simulink model "torque_control_motor_sm"  (R2023b)
settings: Solver=FixedStepAuto  StartTime=0.0  StopTime=inf  RelTol=1e-3  EnableMultiTasking=on
undefined symbols (not defined in the file): G_v
libraries: mbedblockslib x6, cstblocks x3, stm_qeplib x1
settings Model: ExtModeTrigDuration=10  Creator=miche  LastModifiedBy=miche
settings OptimizationCC: EnhancedBackFolding=on  PassReuseOutputArgsAs=Individual arguments  ZeroExternalMemoryAtStartup=off  ZeroInternalMemoryAtStartup=off  MaxStackSize=64  OptimizeBlockOrder=speed  DifferentSizesBufferReuse=on  OptimizationCustomize=off  EfficientTunableParamExpr=on
settings DebuggingCC: ParameterTunabilityLossMsg=error
settings HardwareCC: ProdBitPerPointer=32  ProdBitPerSizeT=32  ProdBitPerPtrDiffT=32  ProdLargestAtomicInteger=Long  ProdLargestAtomicFloat=Double  ProdWordSize=32  ProdLongLongMode=on  ProdHWDeviceType=ARM Compatible->ARM Cortex
settings SFSimCC: MATLABDynamicMemAlloc=off
settings RTWCC: Description=Embedded Coder  SystemTargetFile=ert.tlc  HardwareBoard=STM32 Nucleo F401RE  TemplateMakefile=ert_default_tmf  Toolchain=GNU Tools for ARM Embedded Processors
settings CodeAppCC: ForceParamTrailComments=on  IgnoreCustomStorageClasses=off  OperatorAnnotations=on  SimulinkDataObjDesc=on  SFDataObjDesc=on  InsertBlockDesc=on
settings ERTTargetCC: ExtModeTransport=3  ExtModeStaticAlloc=on  ExtModeStaticAllocSize=2000  ExtModeMexFile=ext_xcp  ExtModeIntrfLevel=Level2 - Open

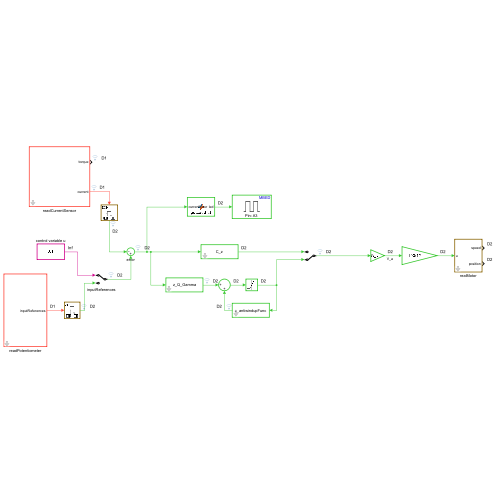
[thumbnail: Simulink's stored preview of the top-level diagram]
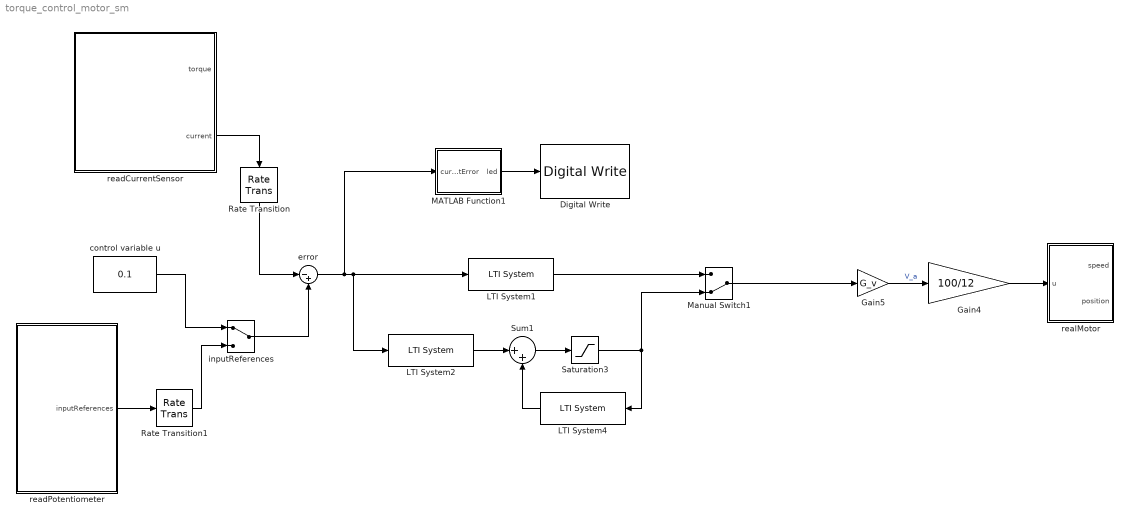
== system torque_control_motor_sm ==
  Digital Write : mbedblockslib/Digital Write  Pin=A3  Direction=output
      settings: LibrarySourceBlock=stmnucleorootlib/Common/Digital Write
  Gain4 : Gain  Gain=100/12
  Gain5 : Gain  Gain=G_v
  LTI System1 : cstblocks/LTI System  sys=C_z  IC=[]  PadeOrder=0
  LTI System2 : cstblocks/LTI System  sys=z_Q_Gamma  IC=[]  PadeOrder=0
  LTI System4 : cstblocks/LTI System  sys=z_antiwindupFunc  IC=[]  PadeOrder=0
  MATLAB Function1 : MATLAB Function  TreatAsAtomicUnit=on
  Manual Switch1 : ManualSwitch  CurrentSetting=0
  Rate Transition : RateTransition
  Rate Transition1 : RateTransition
  Saturation3 : Saturate  UpperLimit=12  LowerLimit=-12
  Sum1 : Sum  Inputs=|++
  control variable u : Constant  Value=0.1
  error : Sum  Inputs=|-+
  inputReferences : ManualSwitch
  readCurrentSensor : Subsystem  mask{alpha=0.9}
  readPotentiometer : Subsystem  mask{alpha=0.9}
  realMotor : Subsystem  mask{Ts=0.005}
      mask prompts: Ts "sample_time"
  wires:
  Gain5/1 -> Gain4/1  "V_a"
  inputReferences/1 -> error/2
  error/1 -> MATLAB Function1/1(currentError), LTI System2/1, LTI System1/1
  MATLAB Function1/1(led) -> Digital Write/1
  control variable u/1 -> inputReferences/1
  Gain4/1 -> realMotor/1(u)
  readPotentiometer/1(inputReferences) -> Rate Transition1/1
  readCurrentSensor/2(current) -> Rate Transition/1
  LTI System4/1 -> Sum1/2
  Saturation3/1 -> LTI System4/1, Manual Switch1/2
  LTI System2/1 -> Sum1/1
  Manual Switch1/1 -> Gain5/1
  Sum1/1 -> Saturation3/1
  LTI System1/1 -> Manual Switch1/1
  Rate Transition/1 -> error/1
  Rate Transition1/1 -> inputReferences/2

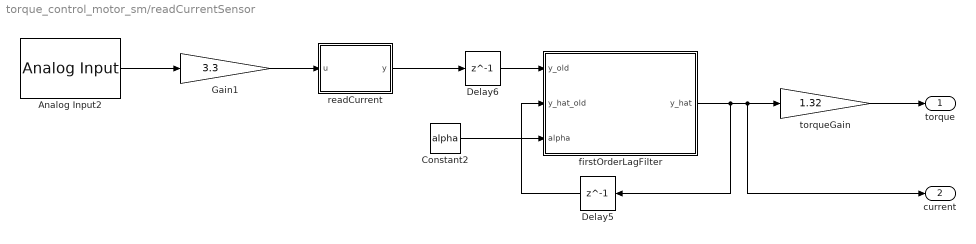
== system torque_control_motor_sm/readCurrentSensor ==
  Analog Input2 : mbedblockslib/Analog Input  Pin=A5  ReadResultsOnly=off  ConversionTriggerSource=Software  ExternalTriggerType=uint32( 0 )  OutputDataType=double  EnableConversionCompleteNotify=off  EnableOuputStatus=off  SampleTime=0.005/20
      settings: LibrarySourceBlock=stmnucleorootlib/Common/Analog Input
  Constant2 : Constant  Value=alpha
  Delay5 : Delay  DelayLength=1  InitialCondition=0
  Delay6 : Delay  DelayLength=1  InitialCondition=0
  Gain1 : Gain  Gain=3.3
  firstOrderLagFilter : MATLAB Function  TreatAsAtomicUnit=on
  readCurrent : MATLAB Function  TreatAsAtomicUnit=on
  torqueGain : Gain  Gain=1.32
  torque : Outport
  current : Outport  Port=2
  wires:
  Constant2/1 -> firstOrderLagFilter/3(alpha)
  firstOrderLagFilter/1(y_hat) -> current/1, torqueGain/1, Delay5/1
  torqueGain/1 -> torque/1
  Gain1/1 -> readCurrent/1(u)
  Analog Input2/1 -> Gain1/1
  readCurrent/1(y) -> Delay6/1
  Delay5/1 -> firstOrderLagFilter/2(y_hat_old)
  Delay6/1 -> firstOrderLagFilter/1(y_old)

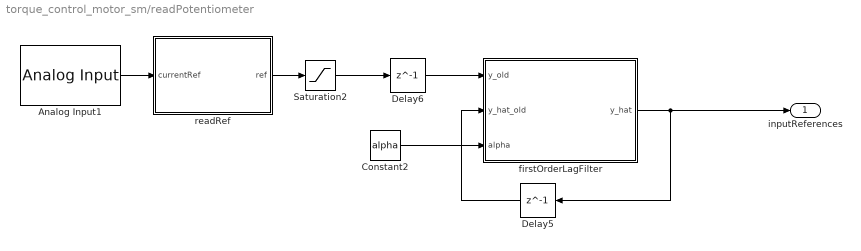
== system torque_control_motor_sm/readPotentiometer ==
  Analog Input1 : mbedblockslib/Analog Input  Pin=A4  ReadResultsOnly=off  ConversionTriggerSource=Software  ExternalTriggerType=uint32( 0 )  OutputDataType=double  EnableConversionCompleteNotify=off  EnableOuputStatus=off  SampleTime=0.005/20
      settings: LibrarySourceBlock=stmnucleorootlib/Common/Analog Input
  Constant2 : Constant  Value=alpha
  Delay5 : Delay  DelayLength=1  InitialCondition=0
  Delay6 : Delay  DelayLength=1  InitialCondition=0
  Saturation2 : Saturate  UpperLimit=0.25  LowerLimit=0
  firstOrderLagFilter : MATLAB Function  TreatAsAtomicUnit=on
  readRef : MATLAB Function  TreatAsAtomicUnit=on
  inputReferences : Outport
  wires:
  Saturation2/1 -> Delay6/1
  Delay6/1 -> firstOrderLagFilter/1(y_old)
  readRef/1(ref) -> Saturation2/1
  Constant2/1 -> firstOrderLagFilter/3(alpha)
  Delay5/1 -> firstOrderLagFilter/2(y_hat_old)
  firstOrderLagFilter/1(y_hat) -> inputReferences/1, Delay5/1
  Analog Input1/1 -> readRef/1(currentRef)

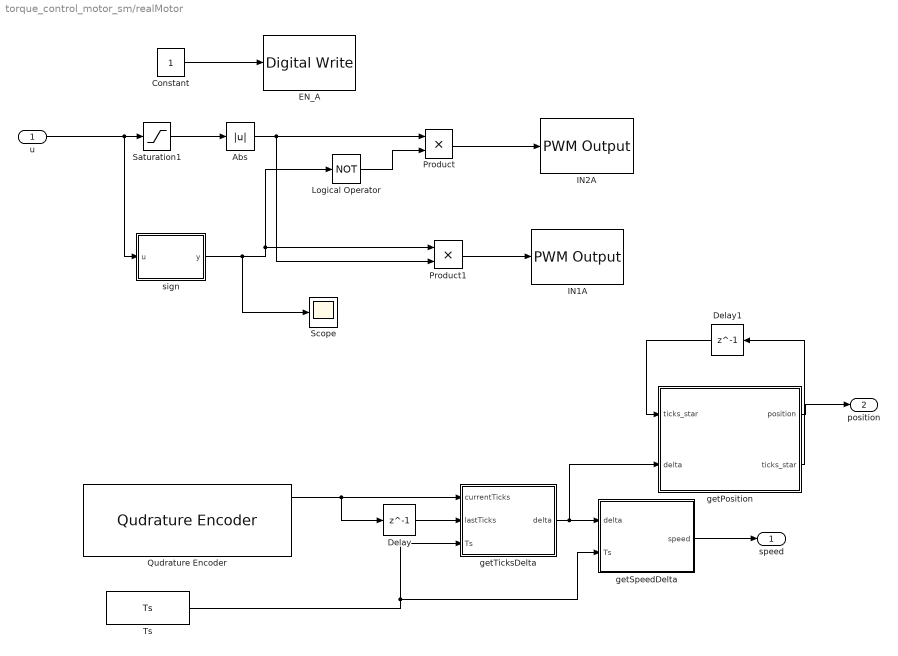
== system torque_control_motor_sm/realMotor ==
  u : Inport
  Abs : Abs  SaturateOnIntegerOverflow=off
  Constant : Constant
  Delay : Delay  DelayLength=1  InitialCondition=0
  Delay1 : Delay  DelayLength=1  InitialCondition=0
  EN_A : mbedblockslib/Digital Write  Pin=2  Direction=output
      settings: LibrarySourceBlock=stmnucleorootlib/Common/Digital Write
  IN1A : mbedblockslib/PWM Output  Pin=5  EnableInputFrequency=off  InitialFrequency=2000  InitialDutyCycle=50  NotificationType=None
      settings: LibrarySourceBlock=stmnucleorootlib/Common/PWM Output
  IN2A : mbedblockslib/PWM Output  Pin=4  EnableInputFrequency=off  InitialFrequency=2000  InitialDutyCycle=50  NotificationType=None
      settings: LibrarySourceBlock=stmnucleorootlib/Common/PWM Output
  Logical Operator : Logic  Operator=NOT  AllPortsSameDT=off  OutDataTypeStr=boolean
  Product : Product
  Product1 : Product
  Qudrature Encoder : stm_qeplib/Qudrature Encoder  SampleTime=0.005
  Saturation1 : Saturate  UpperLimit=100  LowerLimit=-100
  Scope : Scope
  Ts : Constant  Value=Ts
  getPosition : MATLAB Function  TreatAsAtomicUnit=on
  getSpeedDelta : MATLAB Function  TreatAsAtomicUnit=on
  getTicksDelta : MATLAB Function  TreatAsAtomicUnit=on
  sign : MATLAB Function  TreatAsAtomicUnit=on
  speed : Outport
  position : Outport  Port=2
  wires:
  sign/1(y) -> Scope/1, Product1/1, Logical Operator/1
  Ts/1 -> getSpeedDelta/2(Ts), getTicksDelta/3(Ts)
  Qudrature Encoder/1 -> Delay/1, getTicksDelta/1(currentTicks)
  Delay1/1 -> getPosition/1("ticks_star ")
  Constant/1 -> EN_A/1
  getPosition/2(ticks_star) -> Delay1/1
  getTicksDelta/1(delta) -> getPosition/2(delta), getSpeedDelta/1(delta)
  Abs/1 -> Product1/2, Product/1
  Product/1 -> IN2A/1
  Logical Operator/1 -> Product/2
  Product1/1 -> IN1A/1
  Delay/1 -> getTicksDelta/2(lastTicks)
  Saturation1/1 -> Abs/1
  getPosition/1(position) -> position/1
  u/1 -> sign/1(u), Saturation1/1
  getSpeedDelta/1(speed) -> speed/1

== matlab function torque_control_motor_sm/realMotor/getPosition ==
  data: ticks_star input; delta input; position output; ticks_star output
function [position,ticks_star] = getPosition(ticks_star, delta)
    ticks_star=double(ticks_star + delta);
    completeTheta=2*pi*ticks_star/(8400);
    position=completeTheta
    %position=sign(completeTheta)*mod(abs(completeTheta), 2*pi)
end

== matlab function torque_control_motor_sm/realMotor/getSpeedDelta ==
  data: delta input; speed output; Ts input
function speed=getSpeedDelta(delta,Ts)
speed=delta * 60/ (8400*Ts);
end

== matlab function torque_control_motor_sm/readCurrentSensor/firstOrderLagFilter ==
  data: y_old input; y_hat output; y_hat_old input; alpha input
function y_hat = firstOrderLagFilter(y_old, y_hat_old, alpha)
    y_hat= (alpha *y_hat_old) + ((1-alpha)* y_old)
end

== matlab function torque_control_motor_sm/readCurrentSensor/readCurrent ==
  data: u input; y output
function y = readCurrent(u)


y=(u-2.5-0.070)/0.185

== matlab function torque_control_motor_sm/MATLAB Function1 ==
  data: currentError input; led output
function led = getLedStat(currentError) 

    if abs(currentError) < 0.03
        led = true;
    else
        led = false;
    end


end

== matlab function torque_control_motor_sm/realMotor/getTicksDelta ==
  data: currentTicks input; delta output; lastTicks input; Ts input
function delta = getTicksDelta(currentTicks,lastTicks, Ts)

currentTicks=double(currentTicks);
lastTicks=double(lastTicks);

if abs(currentTicks -lastTicks) <= ceil(12600*Ts)
    delta= currentTicks - lastTicks;
else
    if lastTicks > currentTicks
        delta= currentTicks + 2^16 -1 - lastTicks;
    else
        delta= currentTicks - 2^16 +1 - lastTicks;
    end
end

end

== matlab function torque_control_motor_sm/realMotor/sign ==
  data: u input; y output
function y = sign(u)
if u >0
    y=1;
else
   y=0;
end

== matlab function torque_control_motor_sm/readPotentiometer/firstOrderLagFilter ==
  data: y_old input; y_hat output; y_hat_old input; alpha input
function y_hat = firstOrderLagFilter(y_old, y_hat_old, alpha)
    y_hat= (alpha *y_hat_old) + ((1-alpha)* y_old)
end

== matlab function torque_control_motor_sm/readPotentiometer/readRef ==
  data: currentRef input; ref output
function ref= getRef(currentRef) 
    
    ref = currentRef * 0.25
end
